simulink model "SMC"  (R2020a)
settings: Solver=FixedStepAuto  StartTime=0.0  StopTime=15  RelTol=1e-3
InitFcn:
  | load motorModel.mat
  | load expsetup
model workspace (MAT data in the model file):
  A = Simulink.Parameter
  A.Value = Simulink.data.Expression
  A.Value.ExpressionString = "[mModel{1,3}.A mModel{2,3}.A mModel{3,3}.A mModel{4,3}.A]"
  A.DataType = 'auto'
  A.Dimensions = -1
  B = Simulink.Parameter
  B.Value = Simulink.data.Expression
  B.Value.ExpressionString = "[mModel{1,3}.B mModel{2,3}.B mModel{3,3}.B mModel{4,3}.B]"
  B.DataType = 'auto'
  B.Dimensions = -1
  C = Simulink.Parameter
  C.Value = Simulink.data.Expression
  C.Value.ExpressionString = "[[c(1) 1]' [c(2) 1]' [c(3) 1]' [c(4) 1]']"
  C.DataType = 'auto'
  C.Dimensions = -1
  SMC_sdosession_filter : sldodialogs.data.SessionData (value not decoded)
  SMC_sdosession_nofilter : sldodialogs.data.SessionData (value not decoded)
  Ts = 0.02
  c = [0.000100000000012 1000 15.849296894 0.222517467365]
  c1 = 0.118600874325
  c2 = 2.91808049594
  c3 = 0.151177759262
  c4 = 0.001
  delta = [334.905939706 0.00100007918146 107.742782528 24.198854991]
  delta1 = 0.00474000985035
  delta2 = 0.00100046349186
  delta3 = 8.72141675896
  delta4 = 0.27430252152
  g = [1 0.00100000791815 0.403254702693 0.984259710831]
  g1 = 0.999899996387
  g2 = 0.965814768853
  g3 = 0.424400112034
  g4 = 0.931566101393
  k_lp = [0.871372660946 0.960753032772 1 1]
  m = [0.0001 0.000100079181457 29.4777330962 507.481683532]
  m1 = 5.91731016144
  m2 = 15.2521339983
  m3 = 0.806447532242
  m4 = 14.3933541964
  q = [1 0.999999992082 0.738889548079 0.999999992129]
  q1 = 0.801320329502
  q2 = 0.00667518808387
  q3 = 0.500113400189
  q4 = 0.999
  tau_lp = [0.0126999999999 0.0127 0.0127000000001 0.0127]
undefined symbols (not defined in the file or in its folder): DiscIntNeverNeededParam, mModel, x607325_PPR
undefined symbols (not defined in the file): k, u_in, X
libraries: eeGeneralControl x4, simulink_extras x2, simulink x1
settings Model: DataDictionary=MotorInfo.sldd  SimulationMode=accelerator  OrderedModelArguments=off  Creator=khoi  LastModifiedBy=khoi

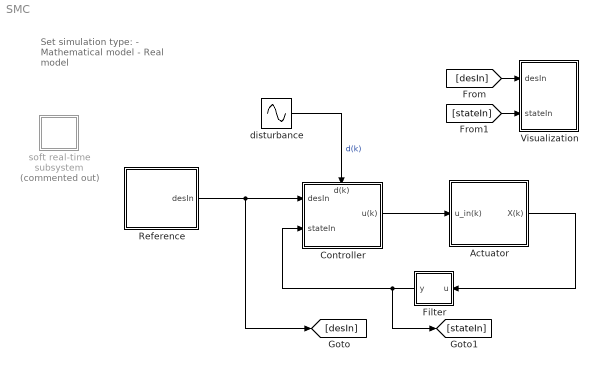
== system SMC ==
  note: Set simulation type:
      | - Mathematical model
      | - Real model
  Actuator : Subsystem
  Controller : Subsystem
      settings: PortSchema="{\"entries\":[{\"content\":{\"sides\":[{\"content\":{\"connectorIds\":[\"In1\",\"In2\"]},\"type\":\"ConnectorPlacement.EquallySpacedRectSide\",\"uuid\":\"ab92a86c-b21c-4625-bceb-c2ca4b22964e\"},{\"content\":{\"connectorIds\":[\"Out1\"],\"side\":\"RIGHT\"},\"type\":\"ConnectorPlacement.EquallySpacedRectSide\",\"uuid\":\"86d5470f-e70b-4cc8-bc91-304fe436d503\"},{\"content\":{\"connectorIds\":[\"In3\"],\"side\":\"TOP\"},\"type\":\"ConnectorPlacement.EquallySpacedRectSide\",\"uuid\":\"909d1e71-533f-4362-b6db-886603c1c7d0\"}]},\"type\":\"ConnectorPlacement.EquallySpacedConnector\",\"uuid\":\"70811cc5-df37-4d12-bd38-ee8baa36081e\"}],\"packageUris\":[\"http://schema.mathworks.com/mf0/Connector/19700101\"],\"version\":\"1.0\"}"
  Filter : Subsystem
  Reference : Subsystem
  Visualization : Subsystem
  disturbance : Sin  Amplitude=1.5  Frequency=2*pi  SampleTime=Ts
  soft real-time subsystem : Subsystem  Commented=on  mask{t_sample=0.01}
      mask prompts: t_sample "Sleep function interval (s)"
  wires:
  Reference/1(desIn) -> Controller/1(desIn), [desIn]
  Controller/1(u(k)) -> Actuator/1(u_in(k))
  Actuator/1(X(k)) -> Filter/1(u)
  Filter/1(y) -> Controller/2(stateIn), [stateIn]
  disturbance/1 -> Controller/3(d(k))  "d(k)"
  [desIn] -> Visualization/1(desIn)
  [stateIn] -> Visualization/2(stateIn)

== system SMC/Actuator ==
  In Bus Element2 : Inport  PortName=u_in(k)  Element=u3(k)
  In Bus Element3 : Inport  PortName=u_in(k)  Element=u4(k)
  In Bus Element4 : Inport  PortName=u_in(k)  Element=u1(k)
  In Bus Element5 : Inport  PortName=u_in(k)  Element=u2(k)
  Variant Subsystem : Subsystem  Variant=on  mask{tfnum=mModel{1,2}.Numerator, tfden=mModel{1,2}.Denominator, NodeID=1, Ts=Ts}
      mask prompts: tfnum "numerator"; tfden "denominaotr"; NodeID "node ID"; Ts "Sample time (s)"
      mask init:
      | myDictionaryObj = Simulink.data.dictionary.open('MotorInfo.sldd');
      mask DialogControl ParameterGroupVar Prompt: Mathematical model
      mask DialogControl ParameterGroupVar_copy Prompt: Mathematical model
  Variant Subsystem1 : Subsystem  Variant=on  mask{tfnum=mModel{2,2}.Numerator, tfden=mModel{2,2}.Denominator, NodeID=2, Ts=Ts}
      mask prompts: tfnum "numerator"; tfden "denominaotr"; NodeID "node ID"; Ts "Sample time (s)"
      mask init:
      | myDictionaryObj = Simulink.data.dictionary.open('MotorInfo.sldd');
      mask DialogControl ParameterGroupVar Prompt: Mathematical model
      mask DialogControl ParameterGroupVar_copy Prompt: Mathematical model
  Variant Subsystem2 : Subsystem  Variant=on  mask{tfnum=mModel{3,2}.Numerator, tfden=mModel{3,2}.Denominator, NodeID=3, Ts=Ts}
      mask prompts: tfnum "numerator"; tfden "denominaotr"; NodeID "node ID"; Ts "Sample time (s)"
      mask init:
      | myDictionaryObj = Simulink.data.dictionary.open('MotorInfo.sldd');
      mask DialogControl ParameterGroupVar Prompt: Mathematical model
      mask DialogControl ParameterGroupVar_copy Prompt: Mathematical model
  Variant Subsystem3 : Subsystem  Variant=on  mask{tfnum=mModel{4,2}.Numerator, tfden=mModel{4,2}.Denominator, NodeID=4, Ts=Ts}
      mask prompts: tfnum "numerator"; tfden "denominaotr"; NodeID "node ID"; Ts "Sample time (s)"
      mask init:
      | myDictionaryObj = Simulink.data.dictionary.open('MotorInfo.sldd');
      mask DialogControl ParameterGroupVar Prompt: Mathematical model
      mask DialogControl ParameterGroupVar_copy Prompt: Mathematical model
  Out Bus Element : Outport  PortName=X(k)  Element=X1
  Out Bus Element1 : Outport  PortName=X(k)  Element=X2
  Out Bus Element2 : Outport  PortName=X(k)  Element=X3
  Out Bus Element3 : Outport  PortName=X(k)  Element=X4
  wires:
  In Bus Element2/1 -> Variant Subsystem/1(u_in(k))
  Variant Subsystem1/1(X(k)) -> Out Bus Element3/1
  Variant Subsystem/1(X(k)) -> Out Bus Element2/1
  Variant Subsystem3/1(X(k)) -> Out Bus Element1/1
  Variant Subsystem2/1(X(k)) -> Out Bus Element/1
  In Bus Element3/1 -> Variant Subsystem1/1(u_in(k))
  In Bus Element4/1 -> Variant Subsystem2/1(u_in(k))
  In Bus Element5/1 -> Variant Subsystem3/1(u_in(k))

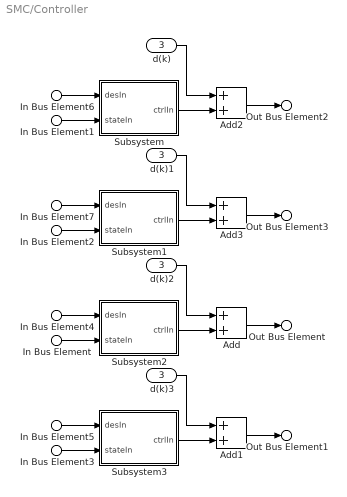
== system SMC/Controller ==
  In Bus Element4 : Inport  PortName=desIn  Element=m1
  In Bus Element5 : Inport  PortName=desIn  Element=m2
  In Bus Element6 : Inport  PortName=desIn  Element=m3
  In Bus Element7 : Inport  PortName=desIn  Element=m4
  In Bus Element : Inport  Port=2  PortName=stateIn  Element=X1
  In Bus Element1 : Inport  Port=2  PortName=stateIn  Element=X3
  In Bus Element2 : Inport  Port=2  PortName=stateIn  Element=X4
  In Bus Element3 : Inport  Port=2  PortName=stateIn  Element=X2
  d(k) : Inport  Port=3
  Add{,1..3} (4 alike) : Sum
  Subsystem : Subsystem  mask{A=mModel{1,3}.A, B=mModel{1,3}.B, C=[c1 1]', g=g1, q=q1, m=m1, delta=delta1, Ts=Ts}
      mask prompts: A "state space A"; B "state space B"; C "state space C"; g "SMC param 1 - g"; q "SMC param 2 - q"; m "SMC param 3 - m"; delta "SMC param 4 - delta"; Ts "Sample time"
  Subsystem1 : Subsystem  mask{A=mModel{2,3}.A, B=mModel{2,3}.B, C=[c2 1]', g=g2, q=q2, m=m2, delta=delta2, Ts=Ts}
      mask prompts: A "state space A"; B "state space B"; C "state space C"; g "SMC param 1 - g"; q "SMC param 2 - q"; m "SMC param 3 - m"; delta "SMC param 4 - delta"; Ts "Sample time"
  Subsystem2 : Subsystem  mask{A=mModel{4,3}.A, B=mModel{4,3}.B, C=[c4 1]', g=g4, q=q4, m=m4, delta=delta4, Ts=Ts}
      mask prompts: A "state space A"; B "state space B"; C "state space C"; g "SMC param 1 - g"; q "SMC param 2 - q"; m "SMC param 3 - m"; delta "SMC param 4 - delta"; Ts "Sample time"
  Subsystem3 : Subsystem  mask{A=mModel{3,3}.A, B=mModel{3,3}.B, C=[c3 1]', g=g3, q=q3, m=m3, delta=delta3, Ts=Ts}
      mask prompts: A "state space A"; B "state space B"; C "state space C"; g "SMC param 1 - g"; q "SMC param 2 - q"; m "SMC param 3 - m"; delta "SMC param 4 - delta"; Ts "Sample time"
  d(k)1 : InportShadow  Port=3
  d(k)2 : InportShadow  Port=3
  d(k)3 : InportShadow  Port=3
  Out Bus Element : Outport  PortName=u(k)  Element=u1(k)
  Out Bus Element1 : Outport  PortName=u(k)  Element=u2(k)
  Out Bus Element2 : Outport  PortName=u(k)  Element=u3(k)
  Out Bus Element3 : Outport  PortName=u(k)  Element=u4(k)
  wires:
  In Bus Element5/1 -> Subsystem3/1(desIn)
  In Bus Element4/1 -> Subsystem2/1(desIn)
  In Bus Element3/1 -> Subsystem3/2(stateIn)
  d(k)1/1 -> Add3/1
  d(k)2/1 -> Add/1
  d(k)/1 -> Add2/1
  In Bus Element/1 -> Subsystem2/2(stateIn)
  In Bus Element7/1 -> Subsystem1/1(desIn)
  In Bus Element2/1 -> Subsystem1/2(stateIn)
  In Bus Element1/1 -> Subsystem/2(stateIn)
  In Bus Element6/1 -> Subsystem/1(desIn)
  Add/1 -> Out Bus Element/1
  d(k)3/1 -> Add1/1
  Add1/1 -> Out Bus Element1/1
  Subsystem1/1(ctrlIn) -> Add3/2
  Subsystem/1(ctrlIn) -> Add2/2
  Add2/1 -> Out Bus Element2/1
  Add3/1 -> Out Bus Element3/1
  Subsystem2/1(ctrlIn) -> Add/2
  Subsystem3/1(ctrlIn) -> Add1/2

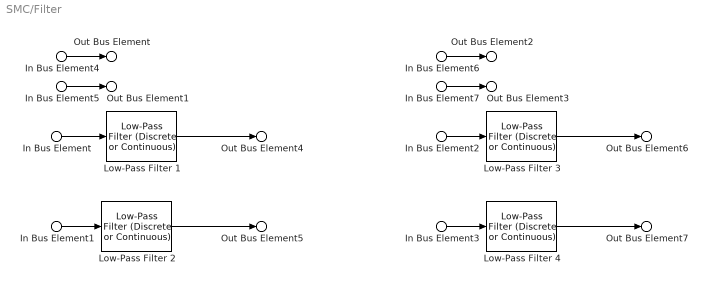
== system SMC/Filter ==
  In Bus Element : Inport  PortName=u  Element=X1.dx(k)
  In Bus Element4 : Inport  PortName=u  Element=X1.x(k)
  In Bus Element1 : Inport  PortName=u  Element=X2.dx(k)
  In Bus Element5 : Inport  PortName=u  Element=X2.x(k)
  In Bus Element2 : Inport  PortName=u  Element=X3.dx(k)
  In Bus Element6 : Inport  PortName=u  Element=X3.x(k)
  In Bus Element3 : Inport  PortName=u  Element=X4.dx(k)
  In Bus Element7 : Inport  PortName=u  Element=X4.x(k)
  Low-Pass Filter 1 : eeGeneralControl/Low-Pass Filter (Discrete or Continuous)  K=k_lp(1)  T=tau_lp(1)  B=inf  A=-inf  init_option=Inherited from block input  x0=0  Ts=-1
  Low-Pass Filter 2 : eeGeneralControl/Low-Pass Filter (Discrete or Continuous)  K=k_lp(2)  T=tau_lp(2)  B=inf  A=-inf  init_option=Inherited from block input  x0=0  Ts=-1
  Low-Pass Filter 3 : eeGeneralControl/Low-Pass Filter (Discrete or Continuous)  K=k_lp(3)  T=tau_lp(3)  B=inf  A=-inf  init_option=Inherited from block input  x0=0  Ts=-1
  Low-Pass Filter 4 : eeGeneralControl/Low-Pass Filter (Discrete or Continuous)  K=k_lp(4)  T=tau_lp(4)  B=inf  A=-inf  init_option=Inherited from block input  x0=0  Ts=-1
  Out Bus Element : Outport  PortName=y  Element=X1.x(k)
  Out Bus Element4 : Outport  PortName=y  Element=X1.dx(k)
  Out Bus Element2 : Outport  PortName=y  Element=X3.x(k)
  Out Bus Element6 : Outport  PortName=y  Element=X3.dx(k)
  Out Bus Element3 : Outport  PortName=y  Element=X4.x(k)
  Out Bus Element7 : Outport  PortName=y  Element=X4.dx(k)
  Out Bus Element1 : Outport  PortName=y  Element=X2.x(k)
  Out Bus Element5 : Outport  PortName=y  Element=X2.dx(k)
  wires:
  Low-Pass Filter 4/1 -> Out Bus Element7/1
  In Bus Element1/1 -> Low-Pass Filter 2/1
  In Bus Element3/1 -> Low-Pass Filter 4/1
  Low-Pass Filter 3/1 -> Out Bus Element6/1
  In Bus Element2/1 -> Low-Pass Filter 3/1
  In Bus Element6/1 -> Out Bus Element2/1
  Low-Pass Filter 2/1 -> Out Bus Element5/1
  In Bus Element5/1 -> Out Bus Element1/1
  In Bus Element7/1 -> Out Bus Element3/1
  In Bus Element4/1 -> Out Bus Element/1
  Low-Pass Filter 1/1 -> Out Bus Element4/1
  In Bus Element/1 -> Low-Pass Filter 1/1

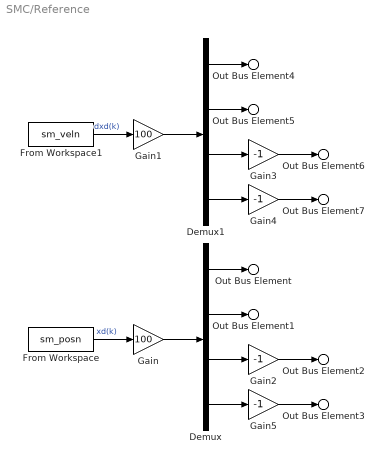
== system SMC/Reference ==
  Demux : Demux
  Demux1 : Demux
  From Workspace : FromWorkspace  VariableName=sm_posn  SampleTime=Ts
  From Workspace1 : FromWorkspace  VariableName=sm_veln  SampleTime=Ts
  Gain : Gain  Gain=100
  Gain1 : Gain  Gain=100
  Gain{2..5} (4 alike) : Gain  Gain=-1
  Out Bus Element : Outport  PortName=desIn  Element=m1.x(k)
  Out Bus Element4 : Outport  PortName=desIn  Element=m1.dx(k)
  Out Bus Element1 : Outport  PortName=desIn  Element=m2.x(k)
  Out Bus Element5 : Outport  PortName=desIn  Element=m2.dx(k)
  Out Bus Element2 : Outport  PortName=desIn  Element=m3.x(k)
  Out Bus Element6 : Outport  PortName=desIn  Element=m3.dx(k)
  Out Bus Element3 : Outport  PortName=desIn  Element=m4.x(k)
  Out Bus Element7 : Outport  PortName=desIn  Element=m4.dx(k)
  wires:
  Gain5/1 -> Out Bus Element3/1
  Gain3/1 -> Out Bus Element6/1
  Demux1/4 -> Gain4/1
  Demux1/2 -> Out Bus Element5/1
  Demux/3 -> Gain2/1
  Gain4/1 -> Out Bus Element7/1
  From Workspace/1 -> Gain/1  "xd(k)"
  Gain1/1 -> Demux1/1
  Demux1/1 -> Out Bus Element4/1
  Gain/1 -> Demux/1
  Demux/4 -> Gain5/1
  Demux1/3 -> Gain3/1
  From Workspace1/1 -> Gain1/1  "dxd(k)"
  Gain2/1 -> Out Bus Element2/1
  Demux/1 -> Out Bus Element/1
  Demux/2 -> Out Bus Element1/1

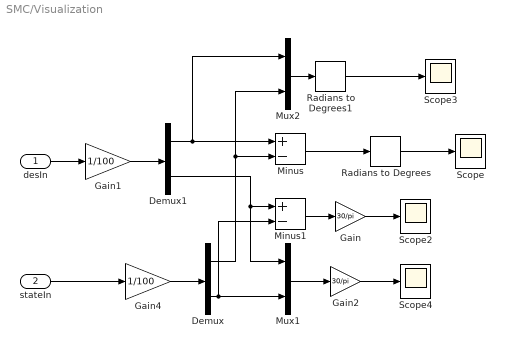
== system SMC/Visualization ==
  desIn : Inport
  stateIn : Inport  Port=2
  Demux : Demux  Outputs=2
  Demux1 : Demux  Outputs=2
  Gain : Gain  Gain=30/pi
  Gain1 : Gain  Gain=1/100
  Gain2 : Gain  Gain=30/pi
  Gain4 : Gain  Gain=1/100
  Minus : Sum  Inputs=+-
  Minus1 : Sum  Inputs=+-
  Mux1 : Mux  Inputs=2
  Mux2 : Mux  Inputs=2
  Radians to Degrees : simulink_extras/Transformations/Radians to Degrees
  Radians to Degrees1 : simulink_extras/Transformations/Radians to Degrees
  Scope{,2..4} (4 alike) : Scope
  wires:
  Mux1/1 -> Gain2/1
  Radians to Degrees1/1 -> Scope3/1
  Demux/1 -> Mux2/2, Minus/2
  Minus1/1 -> Gain/1
  Minus/1 -> Radians to Degrees/1
  Gain4/1 -> Demux/1
  Radians to Degrees/1 -> Scope/1
  Demux1/1 -> Mux2/1, Minus/1
  Mux2/1 -> Radians to Degrees1/1
  Demux1/2 -> Mux1/1, Minus1/1
  stateIn/1 -> Gain4/1
  Demux/2 -> Mux1/2, Minus1/2
  desIn/1 -> Gain1/1
  Gain1/1 -> Demux1/1
  Gain/1 -> Scope2/1
  Gain2/1 -> Scope4/1

== system SMC/soft real-time subsystem ==
  note: What is elapsed real
      | wall-clock time?
  note: What is elapsed
      | simulation time?
  note: Sleep this amount
      | to advance sim time
      | same as wall time
  note: Typically a simple (enough) simulation will fun faster than
      | wall-clock time. This means it's possible for Simulink to
      | simulate, say, 10 seconds in perhps 0.1 or 1 seconds of real
      | wall-clock time.
      |
      | So the challenge is this: how much pause should be inserted
      | every so often to cause the simulation time to advance at
      | the same average rate as real wall-clock time?
      |
      | Using total elapsed time as an absolute reference, this
      | sleep duration will ensure no drift accumulation:
      |
      | t_sleep = t_elapsed_sim_time - t_elapsed_wall_clock_time
      |
      | Pace error and Sleep() or usleep() resolution is system dependent
      | and likely around 10ms on Windows machines. Better on linux.
      |
      | Marc Compere
      | comperem@gmail.com
      | created : 28 May 2018
      | modified: 29 May 2018
      |
      | Reference:
      | Marc Compere (2022). S oft Real Time Block for Pacing Simulink Simulations (https://www.mathworks.com/matlabcentral/fileexchange/67520-soft-real-time-block-for-pacing-simulink-simulations), MATLAB Central File Exchange. Retrieved March 14, 2022.
  Constant : Constant  Value=0
  Display : Display  Commented=on
  MinMax : MinMax  Function=max  Inputs=2
  S-Function : S-Function  FunctionName=sfun_sleep  Parameters=t_sample  SFunctionDeploymentMode=off  EnableBusSupport=off
  Sum : Sum  Inputs=|+-
  get elapsed wall-clock time : Subsystem
  s --> ms : Gain  Gain=1000
  simulation time (s) : Clock
  wires:
  simulation time (s)/1 -> Sum/1
  Constant/1 -> MinMax/2
  get elapsed wall-clock time/1(t_wall_clock_elapsed (s)) -> Sum/2
  Sum/1 -> Display/1, MinMax/1  "pace error (s)"
  MinMax/1 -> s --> ms/1
  s --> ms/1 -> S-Function/1  "sleep duration (ms)"

== system SMC/Actuator/Variant Subsystem ==
  note: 1) Add Subsystem or Model blocks as valid variant choices.
      | 2) You cannot connect blocks at this level. At simulation, connectivity is automatically
      | determined, based on the active variant and port name matching.
  u_in(k) : Inport
  Mathematical model : Subsystem  VariantControl=sim_HIL == false
  Real model : Subsystem  VariantControl=sim_HIL == true
  X(k) : Outport

== system SMC/Actuator/Variant Subsystem1 ==
  note: 1) Add Subsystem or Model blocks as valid variant choices.
      | 2) You cannot connect blocks at this level. At simulation, connectivity is automatically
      | determined, based on the active variant and port name matching.
  u_in(k) : Inport
  Mathematical model : Subsystem  VariantControl=sim_HIL == false
  Real model : Subsystem  VariantControl=sim_HIL == true
  X(k) : Outport

== system SMC/Actuator/Variant Subsystem2 ==
  note: 1) Add Subsystem or Model blocks as valid variant choices.
      | 2) You cannot connect blocks at this level. At simulation, connectivity is automatically
      | determined, based on the active variant and port name matching.
  u_in(k) : Inport
  Mathematical model : Subsystem  VariantControl=sim_HIL == false
  Real model : Subsystem  VariantControl=sim_HIL == true
  X(k) : Outport

== system SMC/Actuator/Variant Subsystem3 ==
  note: 1) Add Subsystem or Model blocks as valid variant choices.
      | 2) You cannot connect blocks at this level. At simulation, connectivity is automatically
      | determined, based on the active variant and port name matching.
  u_in(k) : Inport
  Mathematical model : Subsystem  VariantControl=sim_HIL == false
  Real model : Subsystem  VariantControl=sim_HIL == true
  X(k) : Outport

== system SMC/Controller/Subsystem ==
  desIn : Inport
  stateIn : Inport  Port=2
  Add1 : Sum
  Rate Transition : RateTransition  OutPortSampleTime=Ts
  Subsystem : Subsystem
  Subsystem1 : Subsystem
  ctrlIn : Outport
  wires:
  Subsystem1/2(s(k)) -> Subsystem/1(s(k))
  Subsystem1/1(us(k)) -> Add1/1  "us(k)"
  stateIn/1 -> Subsystem1/2(X(k))  "X(k)"
  Subsystem/1(uc(k)) -> Add1/2  "uc(k)"
  desIn/1 -> Rate Transition/1  "Xd(k)"
  Add1/1 -> ctrlIn/1  "u(k)"
  Rate Transition/1 -> Subsystem1/1(Xd(k))

== system SMC/Controller/Subsystem1 ==
  desIn : Inport
  stateIn : Inport  Port=2
  Add1 : Sum
  Rate Transition : RateTransition  OutPortSampleTime=Ts
  Subsystem : Subsystem
  Subsystem1 : Subsystem
  ctrlIn : Outport
  wires:
  Rate Transition/1 -> Subsystem1/1(Xd(k))
  Add1/1 -> ctrlIn/1  "u(k)"
  desIn/1 -> Rate Transition/1  "Xd(k)"
  Subsystem/1(uc(k)) -> Add1/2  "uc(k)"
  stateIn/1 -> Subsystem1/2(X(k))  "X(k)"
  Subsystem1/1(us(k)) -> Add1/1  "us(k)"
  Subsystem1/2(s(k)) -> Subsystem/1(s(k))

== system SMC/Controller/Subsystem2 ==
  desIn : Inport
  stateIn : Inport  Port=2
  Add1 : Sum
  Rate Transition : RateTransition  OutPortSampleTime=Ts
  Subsystem : Subsystem
  Subsystem1 : Subsystem
  ctrlIn : Outport
  wires:
  Rate Transition/1 -> Subsystem1/1(Xd(k))
  Add1/1 -> ctrlIn/1  "u(k)"
  desIn/1 -> Rate Transition/1  "Xd(k)"
  Subsystem/1(uc(k)) -> Add1/2  "uc(k)"
  stateIn/1 -> Subsystem1/2(X(k))  "X(k)"
  Subsystem1/1(us(k)) -> Add1/1  "us(k)"
  Subsystem1/2(s(k)) -> Subsystem/1(s(k))

== system SMC/Controller/Subsystem3 ==
  desIn : Inport
  stateIn : Inport  Port=2
  Add1 : Sum
  Rate Transition : RateTransition  OutPortSampleTime=Ts
  Subsystem : Subsystem
  Subsystem1 : Subsystem
  ctrlIn : Outport
  wires:
  Subsystem1/2(s(k)) -> Subsystem/1(s(k))
  Subsystem1/1(us(k)) -> Add1/1  "us(k)"
  stateIn/1 -> Subsystem1/2(X(k))  "X(k)"
  Subsystem/1(uc(k)) -> Add1/2  "uc(k)"
  desIn/1 -> Rate Transition/1  "Xd(k)"
  Add1/1 -> ctrlIn/1  "u(k)"
  Rate Transition/1 -> Subsystem1/1(Xd(k))

== system SMC/soft real-time subsystem/get elapsed wall-clock time ==
  note: Block pulled from Mathworks File Exchange entry titled " Raspberry Pi 2, get system clock with timeval "
      |
      | https://www.mathworks.com/matlabcentral/fileexchange/54546-raspberry-pi-2--get-system-clock-with-timeval
  Clock : Clock
  Compare To Zero : simulink/Logic and Bit Operations/Compare To Zero  relop===  OutDataTypeStr=boolean
  S-Function : S-Function  FunctionName=sfun_getSystemClockTimeval  SFunctionDeploymentMode=off  EnableBusSupport=off
  Sum : Sum  Inputs=|+-
  captured value at t==0 : Display  Commented=on
  elapsed wall-clock time (s) (real wall-clock seconds) : Display  Commented=on
  microseconds : Display  Commented=on
  "seconds since January 1st, 1970" : Display  Commented=on
  "seconds since January 1st, 1970 " : Display  Commented=on
  simulation seconds (s) : Display  Commented=on
  triggered capture & hold : Subsystem
  t_wall_clock_elapsed (s) : Outport
  wires:
  triggered capture & hold/1(out) -> captured value at t==0/1, Sum/2
  S-Function/1 -> "seconds since January 1st, 1970 "/1
  Compare To Zero/1 -> triggered capture & hold/2(trigger)
  Sum/1 -> t_wall_clock_elapsed (s)/1, elapsed wall-clock time (s) (real wall-clock seconds)/1
  S-Function/2 -> microseconds/1
  S-Function/3 -> triggered capture & hold/1(value to capture), Sum/1, "seconds since January 1st, 1970"/1
  Clock/1 -> Compare To Zero/1, simulation seconds (s)/1

== system SMC/Actuator/Variant Subsystem/Mathematical model ==
  u_in(k) : Inport
  Discrete-Time Integrator : DiscreteIntegrator  SampleTime=-1  ICPrevOutput=DiscIntNeverNeededParam  ICPrevScaledInput=DiscIntNeverNeededParam
  Rate Transition1 : RateTransition  OutPortSampleTime=Ts
  Transfer Fcn : TransferFcn  Numerator=tfnum  Denominator=tfden
  Zero-Order Hold : ZeroOrderHold  SampleTime=-1
  Out Bus Element : Outport  PortName=X(k)  Element=x(k)
  Out Bus Element1 : Outport  PortName=X(k)  Element=dx(k)
  wires:
  Discrete-Time Integrator/1 -> Out Bus Element/1  "x(k)"
  u_in(k)/1 -> Zero-Order Hold/1
  Zero-Order Hold/1 -> Transfer Fcn/1
  Transfer Fcn/1 -> Rate Transition1/1
  Rate Transition1/1 -> Out Bus Element1/1, Discrete-Time Integrator/1

== system SMC/Actuator/Variant Subsystem/Real model ==
  u_in(k) : Inport
  Bus Selector : BusSelector  OutputSignals=Angle,Speed
  Gain : Gain  Gain=pi/30
  Gain1 : Gain  Gain=30/pi
  Motor 1 : S-Function  FunctionName=sfun_maxon  Parameters=NodeID, DeltaT, OpMode  SFunctionDeploymentMode=off  EnableBusSupport=off  mask{NodeID=NodeID, DeltaT=Ts, OpMode=Cyclic synchronous velocity mode, P_cur=0, I_cur=0, P_pos=0, I_pos=0, D_pos=0, v_posGainFF=0, a_posGainFF=0, P_vel=0, I_vel=0, v_velGainFF=0, a_velGainFF=0, f_velCutoff=0}
      mask prompts: NodeID "Node ID"; DeltaT "Sample time (s)"; OpMode "Operation mode"; P_cur "P gain"; I_cur "I gain"; P_pos "P gain"; I_pos "I gain"; D_pos "D gain"; v_posGainFF "FF velocity gain"; a_posGainFF "FF acceleration gain"; P_vel "P gain"; I_vel "I gain"; v_velGainFF "Feed-forward velocity gain"; a_velGainFF "Feed-forward acceleration gain"; f_velCutoff "Filter cut-off frequency"
      mask TypeOptions OpMode: Cyclic synchronous current (torque) mode | Cyclic synchronous velocity mode | Cyclic synchronous position mode | Profile velocity mode | Profile position mode
      mask DialogControl DescGroupVar Prompt: Motor Parameters
      mask DialogControl DescTextVar Prompt: The block outputs MotorInfo bus signal, which consists of the following variables: angle (increment), speed (rpm), current (mA)
      mask DialogControl Container6 Prompt: Motor
      mask DialogControl Container14 Prompt: Controller Parameters
      mask DialogControl DescTextVar_copy Prompt: This tab is experimental and does not implemented yet. Changing these parameters will not affect the motor performance.
      mask DialogControl Container15 Prompt: Current controller parameter set
      mask DialogControl Container15_copy Prompt: Position controller parameter set
      mask DialogControl Container15_copy_copy Prompt: Velocity controller parameter set
      mask Display:
      | disp('Maxon motor\nHIL');
      | % port_label('input', 1, 'inputSignal');
      | % port_label('output', 1, 'SENSR');
  Rate Transition1 : RateTransition
  Zero-Order Hold : ZeroOrderHold  SampleTime=-1
  rev to rad : Gain  Gain=2*pi/x607325_PPR
  Out Bus Element : Outport  PortName=X(k)  Element=x
  Out Bus Element1 : Outport  PortName=X(k)  Element=dx
  wires:
  Gain/1 -> Out Bus Element1/1
  u_in(k)/1 -> Zero-Order Hold/1
  Zero-Order Hold/1 -> Gain1/1
  Rate Transition1/1 -> Bus Selector/1
  Motor 1/1 -> Rate Transition1/1  "sensorFeedback"
  rev to rad/1 -> Out Bus Element/1
  Gain1/1 -> Motor 1/1
  Bus Selector/1 -> rev to rad/1  "<Angle>"
  Bus Selector/2 -> Gain/1  "<Speed>"

== system SMC/Actuator/Variant Subsystem1/Mathematical model ==
  u_in(k) : Inport
  Discrete-Time Integrator : DiscreteIntegrator  SampleTime=-1  ICPrevOutput=DiscIntNeverNeededParam  ICPrevScaledInput=DiscIntNeverNeededParam
  Rate Transition1 : RateTransition  OutPortSampleTime=Ts
  Transfer Fcn : TransferFcn  Numerator=tfnum  Denominator=tfden
  Zero-Order Hold : ZeroOrderHold  SampleTime=-1
  Out Bus Element : Outport  PortName=X(k)  Element=x(k)
  Out Bus Element1 : Outport  PortName=X(k)  Element=dx(k)
  wires:
  Rate Transition1/1 -> Discrete-Time Integrator/1, Out Bus Element1/1
  Transfer Fcn/1 -> Rate Transition1/1
  Zero-Order Hold/1 -> Transfer Fcn/1
  u_in(k)/1 -> Zero-Order Hold/1
  Discrete-Time Integrator/1 -> Out Bus Element/1  "x(k)"

== system SMC/Actuator/Variant Subsystem1/Real model ==
  u_in(k) : Inport
  Bus Selector : BusSelector  OutputSignals=Angle,Speed
  Gain : Gain  Gain=pi/30
  Gain1 : Gain  Gain=30/pi
  Motor 1 : S-Function  FunctionName=sfun_maxon  Parameters=NodeID, DeltaT, OpMode  SFunctionDeploymentMode=off  EnableBusSupport=off  mask{NodeID=NodeID, DeltaT=Ts, OpMode=Cyclic synchronous velocity mode, P_cur=0, I_cur=0, P_pos=0, I_pos=0, D_pos=0, v_posGainFF=0, a_posGainFF=0, P_vel=0, I_vel=0, v_velGainFF=0, a_velGainFF=0, f_velCutoff=0}
      mask prompts: NodeID "Node ID"; DeltaT "Sample time (s)"; OpMode "Operation mode"; P_cur "P gain"; I_cur "I gain"; P_pos "P gain"; I_pos "I gain"; D_pos "D gain"; v_posGainFF "FF velocity gain"; a_posGainFF "FF acceleration gain"; P_vel "P gain"; I_vel "I gain"; v_velGainFF "Feed-forward velocity gain"; a_velGainFF "Feed-forward acceleration gain"; f_velCutoff "Filter cut-off frequency"
      mask TypeOptions OpMode: Cyclic synchronous current (torque) mode | Cyclic synchronous velocity mode | Cyclic synchronous position mode | Profile velocity mode | Profile position mode
      mask DialogControl DescGroupVar Prompt: Motor Parameters
      mask DialogControl DescTextVar Prompt: The block outputs MotorInfo bus signal, which consists of the following variables: angle (increment), speed (rpm), current (mA)
      mask DialogControl Container6 Prompt: Motor
      mask DialogControl Container14 Prompt: Controller Parameters
      mask DialogControl DescTextVar_copy Prompt: This tab is experimental and does not implemented yet. Changing these parameters will not affect the motor performance.
      mask DialogControl Container15 Prompt: Current controller parameter set
      mask DialogControl Container15_copy Prompt: Position controller parameter set
      mask DialogControl Container15_copy_copy Prompt: Velocity controller parameter set
      mask Display:
      | disp('Maxon motor\nHIL');
      | % port_label('input', 1, 'inputSignal');
      | % port_label('output', 1, 'SENSR');
  Rate Transition1 : RateTransition
  Zero-Order Hold : ZeroOrderHold  SampleTime=-1
  rev to rad : Gain  Gain=2*pi/x607325_PPR
  Out Bus Element : Outport  PortName=X(k)  Element=x
  Out Bus Element1 : Outport  PortName=X(k)  Element=dx
  wires:
  Bus Selector/2 -> Gain/1  "<Speed>"
  Bus Selector/1 -> rev to rad/1  "<Angle>"
  Gain1/1 -> Motor 1/1
  rev to rad/1 -> Out Bus Element/1
  Motor 1/1 -> Rate Transition1/1  "sensorFeedback"
  Rate Transition1/1 -> Bus Selector/1
  Zero-Order Hold/1 -> Gain1/1
  u_in(k)/1 -> Zero-Order Hold/1
  Gain/1 -> Out Bus Element1/1

== system SMC/Actuator/Variant Subsystem2/Mathematical model ==
  u_in(k) : Inport
  Discrete-Time Integrator : DiscreteIntegrator  SampleTime=-1  ICPrevOutput=DiscIntNeverNeededParam  ICPrevScaledInput=DiscIntNeverNeededParam
  Rate Transition1 : RateTransition  OutPortSampleTime=Ts
  Transfer Fcn : TransferFcn  Numerator=tfnum  Denominator=tfden
  Zero-Order Hold : ZeroOrderHold  SampleTime=-1
  Out Bus Element : Outport  PortName=X(k)  Element=x(k)
  Out Bus Element1 : Outport  PortName=X(k)  Element=dx(k)
  wires:
  Discrete-Time Integrator/1 -> Out Bus Element/1  "x(k)"
  u_in(k)/1 -> Zero-Order Hold/1
  Zero-Order Hold/1 -> Transfer Fcn/1
  Transfer Fcn/1 -> Rate Transition1/1
  Rate Transition1/1 -> Out Bus Element1/1, Discrete-Time Integrator/1

== system SMC/Actuator/Variant Subsystem2/Real model ==
  u_in(k) : Inport
  Bus Selector : BusSelector  OutputSignals=Angle,Speed
  Gain : Gain  Gain=pi/30
  Gain1 : Gain  Gain=30/pi
  Motor 1 : S-Function  FunctionName=sfun_maxon  Parameters=NodeID, DeltaT, OpMode  SFunctionDeploymentMode=off  EnableBusSupport=off  mask{NodeID=NodeID, DeltaT=Ts, OpMode=Cyclic synchronous velocity mode, P_cur=0, I_cur=0, P_pos=0, I_pos=0, D_pos=0, v_posGainFF=0, a_posGainFF=0, P_vel=0, I_vel=0, v_velGainFF=0, a_velGainFF=0, f_velCutoff=0}
      mask prompts: NodeID "Node ID"; DeltaT "Sample time (s)"; OpMode "Operation mode"; P_cur "P gain"; I_cur "I gain"; P_pos "P gain"; I_pos "I gain"; D_pos "D gain"; v_posGainFF "FF velocity gain"; a_posGainFF "FF acceleration gain"; P_vel "P gain"; I_vel "I gain"; v_velGainFF "Feed-forward velocity gain"; a_velGainFF "Feed-forward acceleration gain"; f_velCutoff "Filter cut-off frequency"
      mask TypeOptions OpMode: Cyclic synchronous current (torque) mode | Cyclic synchronous velocity mode | Cyclic synchronous position mode | Profile velocity mode | Profile position mode
      mask DialogControl DescGroupVar Prompt: Motor Parameters
      mask DialogControl DescTextVar Prompt: The block outputs MotorInfo bus signal, which consists of the following variables: angle (increment), speed (rpm), current (mA)
      mask DialogControl Container6 Prompt: Motor
      mask DialogControl Container14 Prompt: Controller Parameters
      mask DialogControl DescTextVar_copy Prompt: This tab is experimental and does not implemented yet. Changing these parameters will not affect the motor performance.
      mask DialogControl Container15 Prompt: Current controller parameter set
      mask DialogControl Container15_copy Prompt: Position controller parameter set
      mask DialogControl Container15_copy_copy Prompt: Velocity controller parameter set
      mask Display:
      | disp('Maxon motor\nHIL');
      | % port_label('input', 1, 'inputSignal');
      | % port_label('output', 1, 'SENSR');
  Rate Transition1 : RateTransition
  Zero-Order Hold : ZeroOrderHold  SampleTime=-1
  rev to rad : Gain  Gain=2*pi/x607325_PPR
  Out Bus Element : Outport  PortName=X(k)  Element=x
  Out Bus Element1 : Outport  PortName=X(k)  Element=dx
  wires:
  Gain/1 -> Out Bus Element1/1
  u_in(k)/1 -> Zero-Order Hold/1
  Zero-Order Hold/1 -> Gain1/1
  Rate Transition1/1 -> Bus Selector/1
  Motor 1/1 -> Rate Transition1/1  "sensorFeedback"
  rev to rad/1 -> Out Bus Element/1
  Gain1/1 -> Motor 1/1
  Bus Selector/1 -> rev to rad/1  "<Angle>"
  Bus Selector/2 -> Gain/1  "<Speed>"

== system SMC/Actuator/Variant Subsystem3/Mathematical model ==
  u_in(k) : Inport
  Discrete-Time Integrator : DiscreteIntegrator  SampleTime=-1  ICPrevOutput=DiscIntNeverNeededParam  ICPrevScaledInput=DiscIntNeverNeededParam
  Rate Transition1 : RateTransition  OutPortSampleTime=Ts
  Transfer Fcn : TransferFcn  Numerator=tfnum  Denominator=tfden
  Zero-Order Hold : ZeroOrderHold  SampleTime=-1
  Out Bus Element : Outport  PortName=X(k)  Element=x(k)
  Out Bus Element1 : Outport  PortName=X(k)  Element=dx(k)
  wires:
  Rate Transition1/1 -> Discrete-Time Integrator/1, Out Bus Element1/1
  Transfer Fcn/1 -> Rate Transition1/1
  Zero-Order Hold/1 -> Transfer Fcn/1
  u_in(k)/1 -> Zero-Order Hold/1
  Discrete-Time Integrator/1 -> Out Bus Element/1  "x(k)"

== system SMC/Actuator/Variant Subsystem3/Real model ==
  u_in(k) : Inport
  Bus Selector : BusSelector  OutputSignals=Angle,Speed
  Gain : Gain  Gain=pi/30
  Gain1 : Gain  Gain=30/pi
  Motor 1 : S-Function  FunctionName=sfun_maxon  Parameters=NodeID, DeltaT, OpMode  SFunctionDeploymentMode=off  EnableBusSupport=off  mask{NodeID=NodeID, DeltaT=Ts, OpMode=Cyclic synchronous velocity mode, P_cur=0, I_cur=0, P_pos=0, I_pos=0, D_pos=0, v_posGainFF=0, a_posGainFF=0, P_vel=0, I_vel=0, v_velGainFF=0, a_velGainFF=0, f_velCutoff=0}
      mask prompts: NodeID "Node ID"; DeltaT "Sample time (s)"; OpMode "Operation mode"; P_cur "P gain"; I_cur "I gain"; P_pos "P gain"; I_pos "I gain"; D_pos "D gain"; v_posGainFF "FF velocity gain"; a_posGainFF "FF acceleration gain"; P_vel "P gain"; I_vel "I gain"; v_velGainFF "Feed-forward velocity gain"; a_velGainFF "Feed-forward acceleration gain"; f_velCutoff "Filter cut-off frequency"
      mask TypeOptions OpMode: Cyclic synchronous current (torque) mode | Cyclic synchronous velocity mode | Cyclic synchronous position mode | Profile velocity mode | Profile position mode
      mask DialogControl DescGroupVar Prompt: Motor Parameters
      mask DialogControl DescTextVar Prompt: The block outputs MotorInfo bus signal, which consists of the following variables: angle (increment), speed (rpm), current (mA)
      mask DialogControl Container6 Prompt: Motor
      mask DialogControl Container14 Prompt: Controller Parameters
      mask DialogControl DescTextVar_copy Prompt: This tab is experimental and does not implemented yet. Changing these parameters will not affect the motor performance.
      mask DialogControl Container15 Prompt: Current controller parameter set
      mask DialogControl Container15_copy Prompt: Position controller parameter set
      mask DialogControl Container15_copy_copy Prompt: Velocity controller parameter set
      mask Display:
      | disp('Maxon motor\nHIL');
      | % port_label('input', 1, 'inputSignal');
      | % port_label('output', 1, 'SENSR');
  Rate Transition1 : RateTransition
  Zero-Order Hold : ZeroOrderHold  SampleTime=-1
  rev to rad : Gain  Gain=2*pi/x607325_PPR
  Out Bus Element : Outport  PortName=X(k)  Element=x
  Out Bus Element1 : Outport  PortName=X(k)  Element=dx
  wires:
  Bus Selector/2 -> Gain/1  "<Speed>"
  Bus Selector/1 -> rev to rad/1  "<Angle>"
  Gain1/1 -> Motor 1/1
  rev to rad/1 -> Out Bus Element/1
  Motor 1/1 -> Rate Transition1/1  "sensorFeedback"
  Rate Transition1/1 -> Bus Selector/1
  Zero-Order Hold/1 -> Gain1/1
  u_in(k)/1 -> Zero-Order Hold/1
  Gain/1 -> Out Bus Element1/1

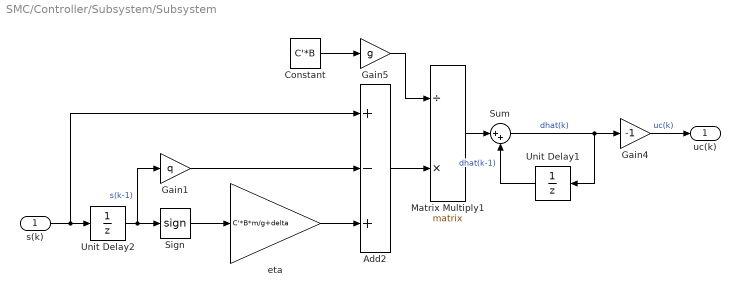
== system SMC/Controller/Subsystem/Subsystem ==
  s(k) : Inport
  Add2 : Sum  Inputs=+-+
  Constant : Constant  Value=C'*B
  Gain1 : Gain  Gain=q
  Gain4 : Gain  Gain=-1
  Gain5 : Gain  Gain=g
  Matrix Multiply1 : Product  Inputs=/*  Multiplication=Matrix(*)
  Sign : Signum
  Sum : Sum  Inputs=|++
  Unit Delay1 : UnitDelay  SampleTime=-1  HasFrameUpgradeWarning=on
  Unit Delay2 : UnitDelay  SampleTime=-1  HasFrameUpgradeWarning=on
  eta : Gain  Gain=C'*B*m/g+delta
  uc(k) : Outport
  wires:
  Add2/1 -> Matrix Multiply1/2
  Constant/1 -> Gain5/1
  Gain1/1 -> Add2/2
  Gain4/1 -> uc(k)/1  "uc(k)"
  Gain5/1 -> Matrix Multiply1/1
  Unit Delay1/1 -> Sum/2  "dhat(k-1)"
  Matrix Multiply1/1 -> Sum/1
  Sum/1 -> Unit Delay1/1, Gain4/1  "dhat(k)"
  Sign/1 -> eta/1
  eta/1 -> Add2/3
  s(k)/1 -> Add2/1, Unit Delay2/1
  Unit Delay2/1 -> Sign/1, Gain1/1  "s(k-1)"

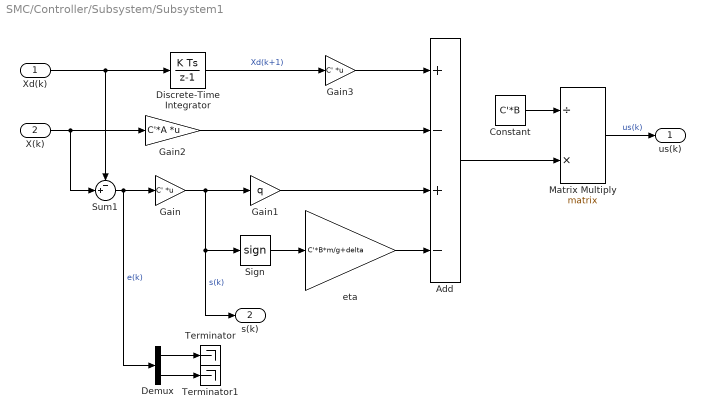
== system SMC/Controller/Subsystem/Subsystem1 ==
  Xd(k) : Inport
  X(k) : Inport  Port=2  PortDimensions=2
  Add : Sum  Inputs=+-+-
  Constant : Constant  Value=C'*B
  Demux : Demux  Outputs=2
  Discrete-Time Integrator : DiscreteIntegrator  SampleTime=-1  ICPrevOutput=DiscIntNeverNeededParam  ICPrevScaledInput=DiscIntNeverNeededParam
  Gain : Gain  Gain=C'  Multiplication=Matrix(K*u)
  Gain1 : Gain  Gain=q
  Gain2 : Gain  Gain=C'*A  Multiplication=Matrix(K*u)
  Gain3 : Gain  Gain=C'  Multiplication=Matrix(K*u)
  Matrix Multiply : Product  Inputs=/*  Multiplication=Matrix(*)
  Sign : Signum
  Sum1 : Sum  Inputs=-+|
  Terminator : Terminator
  Terminator1 : Terminator
  eta : Gain  Gain=C'*B*m/g+delta
  us(k) : Outport
  s(k) : Outport  Port=2
  wires:
  Sign/1 -> eta/1
  Matrix Multiply/1 -> us(k)/1  "us(k)"
  eta/1 -> Add/4
  Gain2/1 -> Add/2
  Sum1/1 -> Demux/1, Gain/1  "e(k)"
  Constant/1 -> Matrix Multiply/1
  Gain1/1 -> Add/3
  Gain3/1 -> Add/1
  Add/1 -> Matrix Multiply/2
  Xd(k)/1 -> Sum1/1, Discrete-Time Integrator/1
  X(k)/1 -> Gain2/1, Sum1/2
  Gain/1 -> Sign/1, s(k)/1, Gain1/1  "s(k)"
  Discrete-Time Integrator/1 -> Gain3/1  "Xd(k+1)"
  Demux/1 -> Terminator/1
  Demux/2 -> Terminator1/1

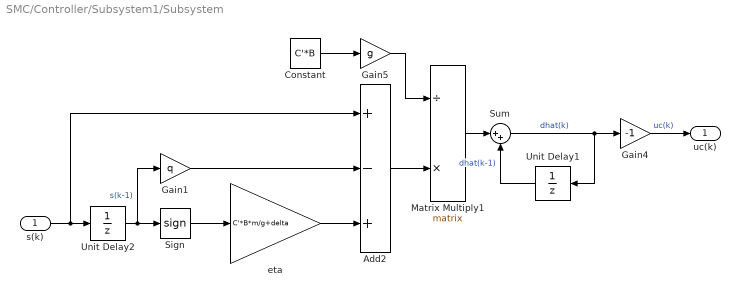
== system SMC/Controller/Subsystem1/Subsystem ==
  s(k) : Inport
  Add2 : Sum  Inputs=+-+
  Constant : Constant  Value=C'*B
  Gain1 : Gain  Gain=q
  Gain4 : Gain  Gain=-1
  Gain5 : Gain  Gain=g
  Matrix Multiply1 : Product  Inputs=/*  Multiplication=Matrix(*)
  Sign : Signum
  Sum : Sum  Inputs=|++
  Unit Delay1 : UnitDelay  SampleTime=-1  HasFrameUpgradeWarning=on
  Unit Delay2 : UnitDelay  SampleTime=-1  HasFrameUpgradeWarning=on
  eta : Gain  Gain=C'*B*m/g+delta
  uc(k) : Outport
  wires:
  Unit Delay2/1 -> Gain1/1, Sign/1  "s(k-1)"
  s(k)/1 -> Unit Delay2/1, Add2/1
  eta/1 -> Add2/3
  Sign/1 -> eta/1
  Sum/1 -> Gain4/1, Unit Delay1/1  "dhat(k)"
  Matrix Multiply1/1 -> Sum/1
  Unit Delay1/1 -> Sum/2  "dhat(k-1)"
  Gain5/1 -> Matrix Multiply1/1
  Gain4/1 -> uc(k)/1  "uc(k)"
  Gain1/1 -> Add2/2
  Constant/1 -> Gain5/1
  Add2/1 -> Matrix Multiply1/2

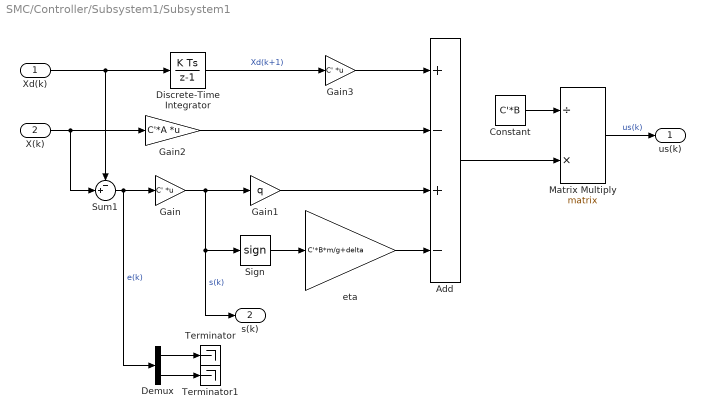
== system SMC/Controller/Subsystem1/Subsystem1 ==
  Xd(k) : Inport
  X(k) : Inport  Port=2  PortDimensions=2
  Add : Sum  Inputs=+-+-
  Constant : Constant  Value=C'*B
  Demux : Demux  Outputs=2
  Discrete-Time Integrator : DiscreteIntegrator  SampleTime=-1  ICPrevOutput=DiscIntNeverNeededParam  ICPrevScaledInput=DiscIntNeverNeededParam
  Gain : Gain  Gain=C'  Multiplication=Matrix(K*u)
  Gain1 : Gain  Gain=q
  Gain2 : Gain  Gain=C'*A  Multiplication=Matrix(K*u)
  Gain3 : Gain  Gain=C'  Multiplication=Matrix(K*u)
  Matrix Multiply : Product  Inputs=/*  Multiplication=Matrix(*)
  Sign : Signum
  Sum1 : Sum  Inputs=-+|
  Terminator : Terminator
  Terminator1 : Terminator
  eta : Gain  Gain=C'*B*m/g+delta
  us(k) : Outport
  s(k) : Outport  Port=2
  wires:
  Demux/2 -> Terminator1/1
  Demux/1 -> Terminator/1
  Discrete-Time Integrator/1 -> Gain3/1  "Xd(k+1)"
  Gain/1 -> Gain1/1, s(k)/1, Sign/1  "s(k)"
  X(k)/1 -> Sum1/2, Gain2/1
  Xd(k)/1 -> Discrete-Time Integrator/1, Sum1/1
  Add/1 -> Matrix Multiply/2
  Gain3/1 -> Add/1
  Gain1/1 -> Add/3
  Constant/1 -> Matrix Multiply/1
  Sum1/1 -> Gain/1, Demux/1  "e(k)"
  Gain2/1 -> Add/2
  eta/1 -> Add/4
  Matrix Multiply/1 -> us(k)/1  "us(k)"
  Sign/1 -> eta/1

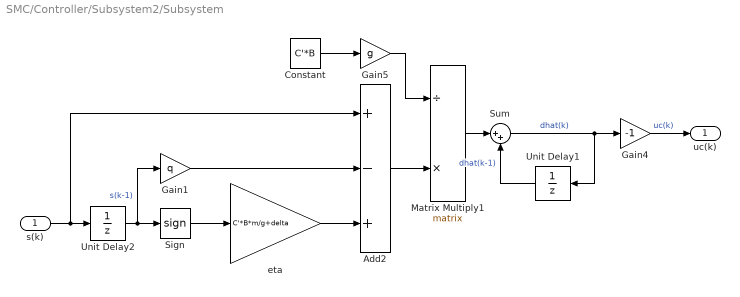
== system SMC/Controller/Subsystem2/Subsystem ==
  s(k) : Inport
  Add2 : Sum  Inputs=+-+
  Constant : Constant  Value=C'*B
  Gain1 : Gain  Gain=q
  Gain4 : Gain  Gain=-1
  Gain5 : Gain  Gain=g
  Matrix Multiply1 : Product  Inputs=/*  Multiplication=Matrix(*)
  Sign : Signum
  Sum : Sum  Inputs=|++
  Unit Delay1 : UnitDelay  SampleTime=-1  HasFrameUpgradeWarning=on
  Unit Delay2 : UnitDelay  SampleTime=-1  HasFrameUpgradeWarning=on
  eta : Gain  Gain=C'*B*m/g+delta
  uc(k) : Outport
  wires:
  Unit Delay2/1 -> Gain1/1, Sign/1  "s(k-1)"
  s(k)/1 -> Unit Delay2/1, Add2/1
  eta/1 -> Add2/3
  Sign/1 -> eta/1
  Sum/1 -> Gain4/1, Unit Delay1/1  "dhat(k)"
  Matrix Multiply1/1 -> Sum/1
  Unit Delay1/1 -> Sum/2  "dhat(k-1)"
  Gain5/1 -> Matrix Multiply1/1
  Gain4/1 -> uc(k)/1  "uc(k)"
  Gain1/1 -> Add2/2
  Constant/1 -> Gain5/1
  Add2/1 -> Matrix Multiply1/2

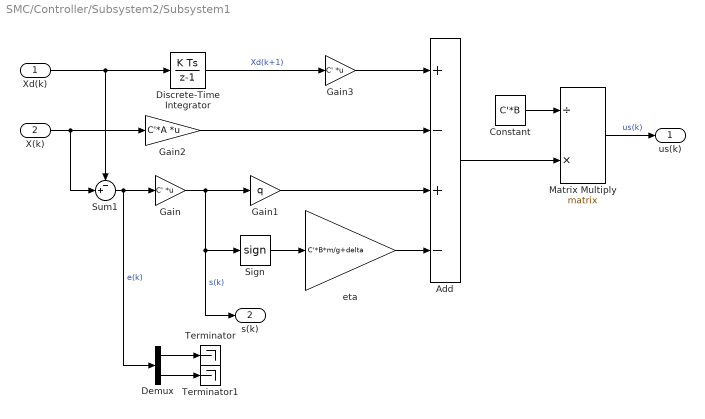
== system SMC/Controller/Subsystem2/Subsystem1 ==
  Xd(k) : Inport
  X(k) : Inport  Port=2  PortDimensions=2
  Add : Sum  Inputs=+-+-
  Constant : Constant  Value=C'*B
  Demux : Demux  Outputs=2
  Discrete-Time Integrator : DiscreteIntegrator  SampleTime=-1  ICPrevOutput=DiscIntNeverNeededParam  ICPrevScaledInput=DiscIntNeverNeededParam
  Gain : Gain  Gain=C'  Multiplication=Matrix(K*u)
  Gain1 : Gain  Gain=q
  Gain2 : Gain  Gain=C'*A  Multiplication=Matrix(K*u)
  Gain3 : Gain  Gain=C'  Multiplication=Matrix(K*u)
  Matrix Multiply : Product  Inputs=/*  Multiplication=Matrix(*)
  Sign : Signum
  Sum1 : Sum  Inputs=-+|
  Terminator : Terminator
  Terminator1 : Terminator
  eta : Gain  Gain=C'*B*m/g+delta
  us(k) : Outport
  s(k) : Outport  Port=2
  wires:
  Demux/2 -> Terminator1/1
  Demux/1 -> Terminator/1
  Discrete-Time Integrator/1 -> Gain3/1  "Xd(k+1)"
  Gain/1 -> Gain1/1, s(k)/1, Sign/1  "s(k)"
  X(k)/1 -> Sum1/2, Gain2/1
  Xd(k)/1 -> Discrete-Time Integrator/1, Sum1/1
  Add/1 -> Matrix Multiply/2
  Gain3/1 -> Add/1
  Gain1/1 -> Add/3
  Constant/1 -> Matrix Multiply/1
  Sum1/1 -> Gain/1, Demux/1  "e(k)"
  Gain2/1 -> Add/2
  eta/1 -> Add/4
  Matrix Multiply/1 -> us(k)/1  "us(k)"
  Sign/1 -> eta/1

== system SMC/Controller/Subsystem3/Subsystem ==
  s(k) : Inport
  Add2 : Sum  Inputs=+-+
  Constant : Constant  Value=C'*B
  Gain1 : Gain  Gain=q
  Gain4 : Gain  Gain=-1
  Gain5 : Gain  Gain=g
  Matrix Multiply1 : Product  Inputs=/*  Multiplication=Matrix(*)
  Sign : Signum
  Sum : Sum  Inputs=|++
  Unit Delay1 : UnitDelay  SampleTime=-1  HasFrameUpgradeWarning=on
  Unit Delay2 : UnitDelay  SampleTime=-1  HasFrameUpgradeWarning=on
  eta : Gain  Gain=C'*B*m/g+delta
  uc(k) : Outport
  wires:
  Add2/1 -> Matrix Multiply1/2
  Constant/1 -> Gain5/1
  Gain1/1 -> Add2/2
  Gain4/1 -> uc(k)/1  "uc(k)"
  Gain5/1 -> Matrix Multiply1/1
  Unit Delay1/1 -> Sum/2  "dhat(k-1)"
  Matrix Multiply1/1 -> Sum/1
  Sum/1 -> Unit Delay1/1, Gain4/1  "dhat(k)"
  Sign/1 -> eta/1
  eta/1 -> Add2/3
  s(k)/1 -> Add2/1, Unit Delay2/1
  Unit Delay2/1 -> Sign/1, Gain1/1  "s(k-1)"

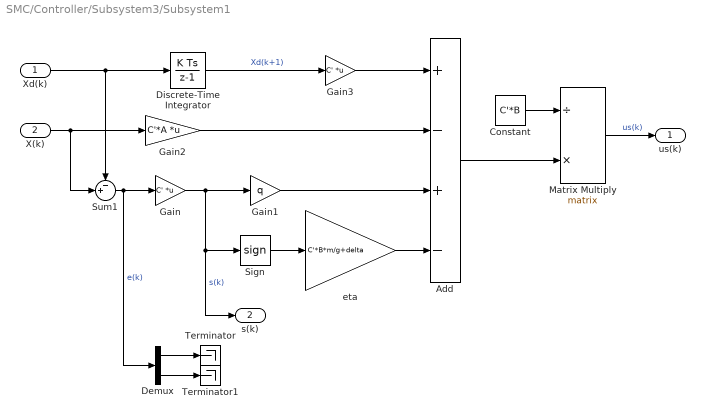
== system SMC/Controller/Subsystem3/Subsystem1 ==
  Xd(k) : Inport
  X(k) : Inport  Port=2  PortDimensions=2
  Add : Sum  Inputs=+-+-
  Constant : Constant  Value=C'*B
  Demux : Demux  Outputs=2
  Discrete-Time Integrator : DiscreteIntegrator  SampleTime=-1  ICPrevOutput=DiscIntNeverNeededParam  ICPrevScaledInput=DiscIntNeverNeededParam
  Gain : Gain  Gain=C'  Multiplication=Matrix(K*u)
  Gain1 : Gain  Gain=q
  Gain2 : Gain  Gain=C'*A  Multiplication=Matrix(K*u)
  Gain3 : Gain  Gain=C'  Multiplication=Matrix(K*u)
  Matrix Multiply : Product  Inputs=/*  Multiplication=Matrix(*)
  Sign : Signum
  Sum1 : Sum  Inputs=-+|
  Terminator : Terminator
  Terminator1 : Terminator
  eta : Gain  Gain=C'*B*m/g+delta
  us(k) : Outport
  s(k) : Outport  Port=2
  wires:
  Sign/1 -> eta/1
  Matrix Multiply/1 -> us(k)/1  "us(k)"
  eta/1 -> Add/4
  Gain2/1 -> Add/2
  Sum1/1 -> Demux/1, Gain/1  "e(k)"
  Constant/1 -> Matrix Multiply/1
  Gain1/1 -> Add/3
  Gain3/1 -> Add/1
  Add/1 -> Matrix Multiply/2
  Xd(k)/1 -> Sum1/1, Discrete-Time Integrator/1
  X(k)/1 -> Gain2/1, Sum1/2
  Gain/1 -> Sign/1, s(k)/1, Gain1/1  "s(k)"
  Discrete-Time Integrator/1 -> Gain3/1  "Xd(k+1)"
  Demux/1 -> Terminator/1
  Demux/2 -> Terminator1/1

== system SMC/soft real-time subsystem/get elapsed wall-clock time/triggered capture & hold ==
  note: Marc Compere
      | comperem@gmail.com
      | created  : 13 September 2002
      | modified: 24 February 2004
  note: if trigger==1,
      |    out(k) = value_to_capture(k)
      | else,
      |    out(k) = out(k-1)
  value to capture : Inport
  trigger : Inport  Port=2
  . : UnitDelay  SampleTime=-1  HasFrameUpgradeWarning=on
  Relational Operator : RelationalOperator  Operator===  RndMeth=Nearest
  Switch : Switch  Threshold=0.5  SaturateOnIntegerOverflow=on
  const : Constant
  out : Outport
  wires:
  trigger/1 -> Relational Operator/1
  const/1 -> Relational Operator/2
  Relational Operator/1 -> Switch/2
  Switch/1 -> ./1, out/1  "out(k)"
  value to capture/1 -> Switch/1
  ./1 -> Switch/3  "out(k-1)"
